simulink model "Lab1__KUKA__IIWA14_corrected"  (R2018b)
settings: Solver=ode4  StartTime=0.0  StopTime=10  FixedStep=0.001  RelTol=1e-3  EnableMultiTasking=on
values from neighbouring files (symbols this model uses):
  q0 = [pi/6; -pi/3; 0; -pi/3; -pi/6; pi/2; pi/2]    [Lab1__KUKA__IIWA14.m]
undefined symbols (not defined in the file or in its folder): v_fun, X, Y, Z
libraries: nesl_utility x41, sm_lib x27
settings Model: Creator=Ramin_hp  LastModifiedBy=Renata
settings OptimizationCC: LifeSpan=inf
settings DebuggingCC: SFUnexpectedBacktrackingDiag=warning  SFNoUnconditionalDefaultTransitionDiag=warning  SFExecutionAtInitializationDiag=none
settings SFSimCC: SimUseLocalCustomCode=off
settings RTWCC: RTWUseLocalCustomCode=off
settings CodeAppCC: StateflowObjectComments=on
settings GRTTargetCC: TargetLangStandard=C89/C90 (ANSI)  GeneratePreprocessorConditionals=Disable all
settings ConfigComp: CovMetricSettings=dw  CovHtmlReporting=on  CovSaveCumulativeToWorkspaceVar=on  CovSaveSingleToWorkspaceVar=on  CovExternalEMLEnable=off
settings SimscapeCC: SimscapeNormalizeSystem=off
settings ExplorerConfigSet: InternalSimMechanicsExplorerSettings="<ExplorerConfiguration><canonicalview>default</canonicalview><AnimationSetting><BasePlaybackSpeed>1.0</BasePlaybackSpeed><PlaybackSpeedFactor>4.0</PlaybackSpeedFactor></AnimationSetting><TilePanel><TileInfo><Tiles Columns=\"2\" Count=\"4\" Rows=\"2\"><Column Weight=\"0.5\"/><Column Weight=\"0.5\"/><Row Weight=\"0.5\"/><Row Weight=\"0.5\"/><Tile Height=\"1\" Width=\"1\" X=\"0\" Y=\"0\"/><Tile Height=\"1\" Width=\"1\" X=\"0\" Y=\"1\"/><Tile Height=\"1\" Width=\"1\" X=\"1\" Y=\"0\"/><Tile Height=\"1\" Width=\"1\" X=\"1\" Y=\"1\"/></Tiles></TileInfo><SceneInfo><SceneViewer><BGColor><R>0.60000002384185791</R><G>0.60000002384185791</G><B>0.60000002384185791</B></BGColor><Camera><DoPerspective>off</DoPerspective><Position><X>-0.162516330727092595</X><Y>-0.986821008184004533</Y><Z>0.680013463560397158</Z></Position><Center><X>-0.162516330727092595</X><Y>0.0131789918159954667</Y><Z>0.680013463560397158</Z></Center><Up><X>0</X><Y>-0</Y><Z>1</Z></Up><ViewLimDist>1</ViewLimDist><YLim>0.631454701364040472</YLim><XLim>1.11901596414291249</XLim></Camera></SceneViewer><SceneViewer><BGColor><R>0.60000002384185791</R><G>0.60000002384185791</G><B>0.60000002384185791</B></BGColor><Camera><DoPerspective>off</DoPerspective><Position><X>-0.37115316295295453</X><Y>-0.0343740496289973579</Y><Z>1.55866333636371568</Z></Position><Center><X>-0.37115316295295453</X><Y>-0.0343740496289973579</Y><Z>0.558663336363715679</Z></Center><Up><X>0</X><Y>1</Y><Z>-0</Z></Up><ViewLimDist>1</ViewLimDist><YLim>0.461610877680944443</YLim><XLim>0.818031665978841804</XLim></Camera></SceneViewer><SceneViewer><BGColor><R>0.60000002384185791</R><G>0.60000002384185791</G><B>0.60000002384185791</B></BGColor><Camera><DoPerspective>off</DoPerspective><Position><X>0.862449510483560777</X><Y>0.0193375746821874417</Y><Z>0.558663276759070793</Z></Position><Center><X>-0.137550489516439223</X><Y>0.0193375746821874417</Y><Z>0.558663276759070793</Z></Center><Up><X>-0</X><Y>0</Y><Z>1</Z></Up><ViewLimDist>1</ViewLimDist><YLim>0.575423637628555307</YLim><XLim>1.01972197730193104</XLim></Camera></SceneViewer><SceneViewer><BGColor><R>0.60000002384185791</R><G>0.60000002384185791</G><B>0.60000002384185791</B></BGColor><Camera><DoPerspective>off</DoPerspective><Position><X>0.430822299974531364</X><Y>-0.567189795663393004</Y><Z>1.10490652072727147</Z></Position><Center><X>-0.169233772465264248</X><Y>0.0328662767764026365</Y><Z>0.504850448287475606</Z></Center><Up><X>-0.408248290463863073</X><Y>0.408248290463863073</Y><Z>0.816496580927726145</Z></Up><ViewLimDist>1</ViewLimDist><YLim>0.611581102013587952</YLim><XLim>1.08379748387806174</XLim></Camera></SceneViewer></SceneInfo></TilePanel><MechEditorPanel><Cameras/><GfxPanelCameraMap/><VideoCreator><PlaybackSpeedRatio>1.0</PlaybackSpeedRatio><FrameRate>30</FrameRate><VideoFormat>Motion JPEG AVI</VideoFormat><FrameSize>auto</FrameSize></VideoCreator></MechEditorPanel></ExplorerConfiguration>"

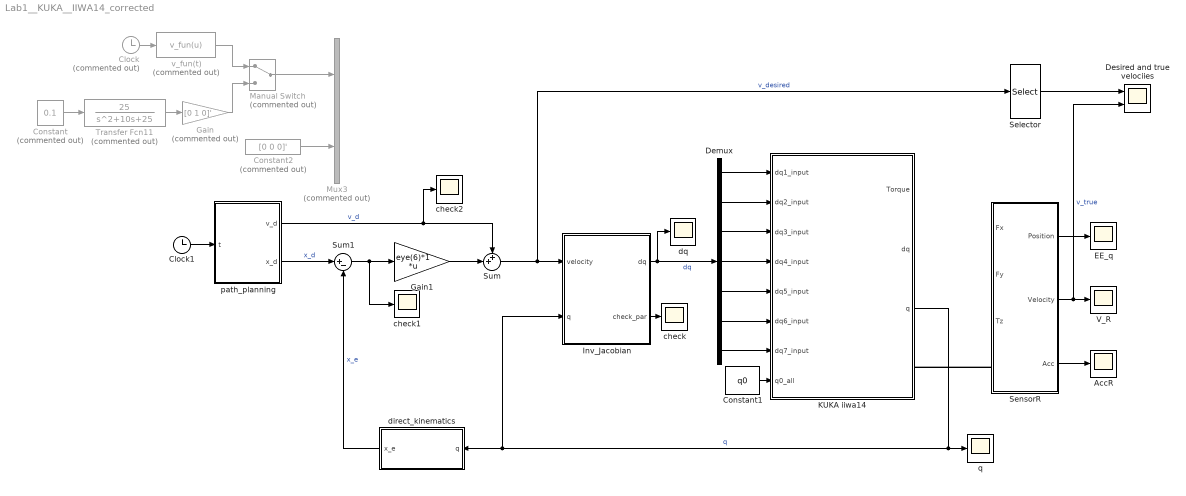
== system Lab1__KUKA__IIWA14_corrected ==
  AccR : Scope
  Clock : Clock  Commented=on
  Clock1 : Clock
  Constant : Constant  Commented=on  Value=0.1
  Constant1 : Constant  Value=q0
  Constant2 : Constant  Commented=on  Value=[0 0 0]'  VectorParams1D=off
  Demux : Demux  Outputs=7
  Desired and true velociies : Scope  NumInputPorts=2
  EE_q : Scope
  Gain : Gain  Commented=on  Gain=[0 1 0]'
  Gain1 : Gain  Gain=eye(6)*1  Multiplication=Matrix(K*u)
  Inv_Jacobian : Subsystem
  KUKA iiwa14 : Subsystem
  Manual Switch : ManualSwitch  Commented=on
  Mux3 : Mux  Commented=on  Inputs=2
  Selector : Selector  InputPortWidth=6  IndexOptions=Index vector (dialog)  Indices=[1 2 3]  OutputSizes=1
  SensorR : Subsystem
  Sum : Sum  Inputs=++|
  Sum1 : Sum  Inputs=|+-
  Transfer Fcn11 : TransferFcn  Commented=on  Numerator=[25]  Denominator=[1 10 25]
  V_R : Scope
  check : Scope
  check1 : Scope
  check2 : Scope
  direct_kinematics : MATLAB Function  TreatAsAtomicUnit=on
  dq : Scope
  path_planning : MATLAB Function  TreatAsAtomicUnit=on
  q : Scope
  v_fun(t) : MATLABFcn  Commented=on  MATLABFcn=v_fun(u)  OutputDimensions=3
  wires:
  Constant1/1 -> KUKA iiwa14/8(q0_all)
  SensorR/2(Velocity) -> Desired and true velociies/2, V_R/1  "v_true"
  SensorR/3(Acc) -> AccR/1
  SensorR/1(Position) -> EE_q/1
  Demux/5 -> KUKA iiwa14/5(dq5_input)
  Demux/4 -> KUKA iiwa14/4(dq4_input)
  Demux/6 -> KUKA iiwa14/6(dq6_input)
  Demux/1 -> KUKA iiwa14/1(dq1_input)
  Demux/2 -> KUKA iiwa14/2(dq2_input)
  Demux/3 -> KUKA iiwa14/3(dq3_input)
  path_planning/1(v_d) -> check2/1, Sum/1  "v_d"
  Demux/7 -> KUKA iiwa14/7(dq7_input)
  Inv_Jacobian/1(dq) -> Demux/1, dq/1  "dq"
  Clock/1 -> v_fun(t)/1
  v_fun(t)/1 -> Manual Switch/1
  Constant/1 -> Transfer Fcn11/1
  Constant2/1 -> Mux3/2
  Transfer Fcn11/1 -> Gain/1
  Gain/1 -> Manual Switch/2
  Manual Switch/1 -> Mux3/1
  Inv_Jacobian/2(check_par) -> check/1
  Sum/1 -> Inv_Jacobian/1(velocity), Selector/1  "v_desired"
  Gain1/1 -> Sum/2
  KUKA iiwa14/3(q) -> Inv_Jacobian/2(q), direct_kinematics/1(q), q/1  "q"
  direct_kinematics/1(x_e) -> Sum1/2  "x_e"
  Sum1/1 -> check1/1, Gain1/1
  path_planning/2(x_d) -> Sum1/1  "x_d"
  Clock1/1 -> path_planning/1(t)
  Selector/1 -> Desired and true velociies/1
  connections:
  SensorR/LConn1 -- KUKA iiwa14/RConn1

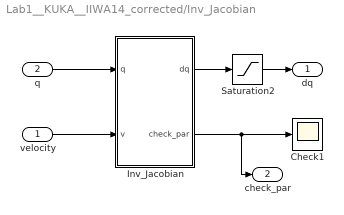
== system Lab1__KUKA__IIWA14_corrected/Inv_Jacobian ==
  velocity : Inport
  q : Inport  Port=2
  Check1 : Scope
  Inv_Jacobian : MATLAB Function  TreatAsAtomicUnit=on
  Saturation2 : Saturate  UpperLimit=9  LowerLimit=-9
  dq : Outport
  check_par : Outport  Port=2
  wires:
  velocity/1 -> Inv_Jacobian/2(v)
  q/1 -> Inv_Jacobian/1(q)
  Saturation2/1 -> dq/1
  Inv_Jacobian/1(dq) -> Saturation2/1
  Inv_Jacobian/2(check_par) -> check_par/1, Check1/1

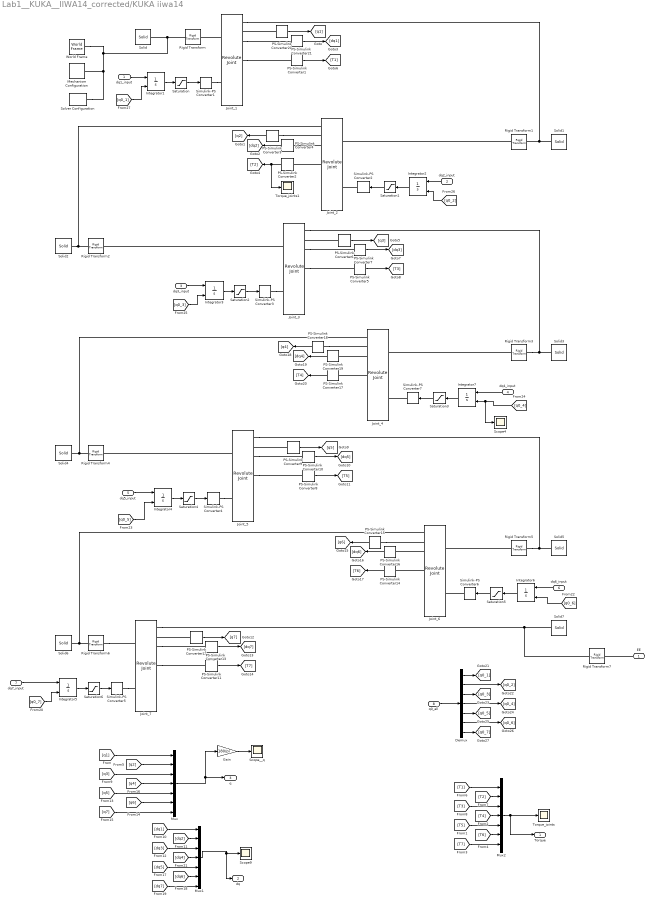
== system Lab1__KUKA__IIWA14_corrected/KUKA iiwa14 ==
  dq1_input : Inport
  dq2_input : Inport  Port=2
  dq3_input : Inport  Port=3
  dq4_input : Inport  Port=4
  dq5_input : Inport  Port=5
  dq6_input : Inport  Port=6
  dq7_input : Inport  Port=7
  q0_all : Inport  Port=8
  Demux : Demux  Outputs=7
  Gain : Gain  Gain=180/pi
  Integrator1 : Integrator  InitialConditionSource=external
  Integrator2 : Integrator  InitialConditionSource=external
  Integrator3 : Integrator  InitialConditionSource=external
  Integrator{4..7} (4 alike) : Integrator  InitialConditionSource=external  InitialCondition=90*pi/180
  Joint_{1..7} (7 alike) : sm_lib/Joints/Revolute Joint  SenseConstraintForce=on  SenseConstraintForceX=off  SenseConstraintForceY=off  SenseConstraintForceZ=off  SenseConstraintTorque=on  SenseConstraintTorqueX=off  SenseConstraintTorqueY=off  SenseConstraintTorqueZ=off  SenseTotalForce=on  SenseTotalForceX=off  SenseTotalForceY=off  SenseTotalForceZ=off  SenseTotalTorque=on  SenseTotalTorqueX=off  SenseTotalTorqueY=off  SenseTotalTorqueZ=off  CompositeWrenchDir=FollowerOnBase  CompositeWrenchFrame=BaseFrame  EquilibriumPosition=0  EquilibriumPositionUnits=deg  SpringStiffness=0  SpringStiffnessUnits=N*m/deg  DampingCoefficient=0.5  DampingCoefficientUnits=N*m/(rad/s)  TorqueActuationMode=ComputedTorque  MotionActuationMode=InputMotion  SensePosition=on  SenseVelocity=on  SenseAcceleration=on  SenseTorqueForce=on  PositionTargetSpecify=off  PositionTargetPriority=High  PositionTargetValue=0  PositionTargetValueUnits=deg  VelocityTargetSpecify=off  VelocityTargetPriority=High  VelocityTargetValue=0  VelocityTargetValueUnits=deg/s
  Mechanism Configuration : sm_lib/Utilities/Mechanism Configuration  UniformGravity=Constant  GravityVector=[0 0 -9.80665]  GravityUnits=m/s^2  LinearizationDelta=0.001
  Mux : Mux  Inputs=7
  Mux1 : Mux  Inputs=7
  Mux2 : Mux  Inputs=7
  PS-Simulink Converter{1..21} (21 alike) : nesl_utility/PS-Simulink Converter  PhysicalDomain=network_engine_domain  SubClassName=ps_output  LeftPortType=input  RightPortType=output  PseudoPeriodic=off  Frequencies=[]  Unit=1  AffineConversion=off
  Rigid Transform : sm_lib/Frames and Transforms/Rigid Transform  TranslationMethod=Cartesian  TranslationStandardOffset=0  TranslationLengthUnit=m  TranslationStandardAxis=+Z  TranslationCartesianOffset=[0 0 0.1575]  TranslationROffset=0  TranslationROffsetUnits=m  TranslationZOffset=0  TranslationZOffsetUnits=m  TranslationThetaOffset=0  TranslationThetaOffsetUnits=deg  RotationMethod=None  RotationAngleUnits=deg  RotationStandardAxis=+Z  RotationAngle=0.0  RotationArbitraryAxis=[0 0 1]  FollAlignAxisA=+X  BaseAlignAxisA=+Y  FollAlignAxisB=+Y  BaseAlignAxisB=+Z  RotationSequenceAxes=FollowerAxes  RotationSequence=XYX  RotationSequenceAngles=[0 0 0]  RotationSequenceAnglesUnits=deg  RotationMatrix=[1 0 0; 0 1 0; 0 0 1]
  Rigid Transform1 : sm_lib/Frames and Transforms/Rigid Transform  TranslationMethod=Cartesian  TranslationStandardOffset=0  TranslationLengthUnit=m  TranslationStandardAxis=+Z  TranslationCartesianOffset=[0 0 0.2025]  TranslationROffset=0  TranslationROffsetUnits=m  TranslationZOffset=0  TranslationZOffsetUnits=m  TranslationThetaOffset=0  TranslationThetaOffsetUnits=deg  RotationMethod=RotationSequence  RotationAngleUnits=deg  RotationStandardAxis=+Z  RotationAngle=0.0  RotationArbitraryAxis=[0 0 1]  FollAlignAxisA=+X  BaseAlignAxisA=+Y  FollAlignAxisB=+Y  BaseAlignAxisB=+Z  RotationSequenceAxes=BaseAxes  RotationSequence=XYZ  RotationSequenceAngles=[pi/2 0 pi]  RotationSequenceAnglesUnits=rad  RotationMatrix=[1 0 0; 0 1 0; 0 0 1]
  Rigid Transform2 : sm_lib/Frames and Transforms/Rigid Transform  TranslationMethod=Cartesian  TranslationStandardOffset=0  TranslationLengthUnit=m  TranslationStandardAxis=+Z  TranslationCartesianOffset=[0 0.2045 0]  TranslationROffset=0  TranslationROffsetUnits=m  TranslationZOffset=0  TranslationZOffsetUnits=m  TranslationThetaOffset=0  TranslationThetaOffsetUnits=deg  RotationMethod=RotationSequence  RotationAngleUnits=deg  RotationStandardAxis=+Z  RotationAngle=0.0  RotationArbitraryAxis=[0 0 1]  FollAlignAxisA=+X  BaseAlignAxisA=+Y  FollAlignAxisB=+Y  BaseAlignAxisB=+Z  RotationSequenceAxes=BaseAxes  RotationSequence=XYZ  RotationSequenceAngles=[pi/2 0 pi]  RotationSequenceAnglesUnits=rad  RotationMatrix=[1 0 0; 0 1 0; 0 0 1]
  Rigid Transform3 : sm_lib/Frames and Transforms/Rigid Transform  TranslationMethod=Cartesian  TranslationStandardOffset=0  TranslationLengthUnit=m  TranslationStandardAxis=+Z  TranslationCartesianOffset=[0 0 0.2155]  TranslationROffset=0  TranslationROffsetUnits=m  TranslationZOffset=0  TranslationZOffsetUnits=m  TranslationThetaOffset=0  TranslationThetaOffsetUnits=deg  RotationMethod=RotationSequence  RotationAngleUnits=deg  RotationStandardAxis=+Z  RotationAngle=0.0  RotationArbitraryAxis=[0 0 1]  FollAlignAxisA=+X  BaseAlignAxisA=+Y  FollAlignAxisB=+Y  BaseAlignAxisB=+Z  RotationSequenceAxes=BaseAxes  RotationSequence=XYZ  RotationSequenceAngles=[pi/2 0 0]  RotationSequenceAnglesUnits=rad  RotationMatrix=[1 0 0; 0 1 0; 0 0 1]
  Rigid Transform4 : sm_lib/Frames and Transforms/Rigid Transform  TranslationMethod=Cartesian  TranslationStandardOffset=0  TranslationLengthUnit=m  TranslationStandardAxis=+Z  TranslationCartesianOffset=[0 0.1845 0]  TranslationROffset=0  TranslationROffsetUnits=m  TranslationZOffset=0  TranslationZOffsetUnits=m  TranslationThetaOffset=0  TranslationThetaOffsetUnits=deg  RotationMethod=RotationSequence  RotationAngleUnits=deg  RotationStandardAxis=+Z  RotationAngle=0.0  RotationArbitraryAxis=[0 0 1]  FollAlignAxisA=+X  BaseAlignAxisA=+Y  FollAlignAxisB=+Y  BaseAlignAxisB=+Z  RotationSequenceAxes=BaseAxes  RotationSequence=XYZ  RotationSequenceAngles=[-pi/2 pi 0]  RotationSequenceAnglesUnits=rad  RotationMatrix=[1 0 0; 0 1 0; 0 0 1]
  Rigid Transform5 : sm_lib/Frames and Transforms/Rigid Transform  TranslationMethod=Cartesian  TranslationStandardOffset=0  TranslationLengthUnit=m  TranslationStandardAxis=+Z  TranslationCartesianOffset=[0 0 0.2155]  TranslationROffset=0  TranslationROffsetUnits=m  TranslationZOffset=0  TranslationZOffsetUnits=m  TranslationThetaOffset=0  TranslationThetaOffsetUnits=deg  RotationMethod=RotationSequence  RotationAngleUnits=deg  RotationStandardAxis=+Z  RotationAngle=0.0  RotationArbitraryAxis=[0 0 1]  FollAlignAxisA=+X  BaseAlignAxisA=+Y  FollAlignAxisB=+Y  BaseAlignAxisB=+Z  RotationSequenceAxes=BaseAxes  RotationSequence=XYZ  RotationSequenceAngles=[pi/2 0 0]  RotationSequenceAnglesUnits=rad  RotationMatrix=[1 0 0; 0 1 0; 0 0 1]
  Rigid Transform6 : sm_lib/Frames and Transforms/Rigid Transform  TranslationMethod=Cartesian  TranslationStandardOffset=0  TranslationLengthUnit=m  TranslationStandardAxis=+Z  TranslationCartesianOffset=[0 0.081 0]  TranslationROffset=0  TranslationROffsetUnits=m  TranslationZOffset=0  TranslationZOffsetUnits=m  TranslationThetaOffset=0  TranslationThetaOffsetUnits=deg  RotationMethod=RotationSequence  RotationAngleUnits=deg  RotationStandardAxis=+Z  RotationAngle=0.0  RotationArbitraryAxis=[0 0 1]  FollAlignAxisA=+X  BaseAlignAxisA=+Y  FollAlignAxisB=+Y  BaseAlignAxisB=+Z  RotationSequenceAxes=BaseAxes  RotationSequence=XYZ  RotationSequenceAngles=[-pi/2 pi 0]  RotationSequenceAnglesUnits=rad  RotationMatrix=[1 0 0; 0 1 0; 0 0 1]
  Rigid Transform7 : sm_lib/Frames and Transforms/Rigid Transform  TranslationMethod=Cartesian  TranslationStandardOffset=0  TranslationLengthUnit=m  TranslationStandardAxis=+Z  TranslationCartesianOffset=[0 0 0.05]  TranslationROffset=0  TranslationROffsetUnits=m  TranslationZOffset=0  TranslationZOffsetUnits=m  TranslationThetaOffset=0  TranslationThetaOffsetUnits=deg  RotationMethod=RotationSequence  RotationAngleUnits=deg  RotationStandardAxis=+Z  RotationAngle=0.0  RotationArbitraryAxis=[0 0 1]  FollAlignAxisA=+X  BaseAlignAxisA=+Y  FollAlignAxisB=+Y  BaseAlignAxisB=+Z  RotationSequenceAxes=BaseAxes  RotationSequence=XYZ  RotationSequenceAngles=[-pi/2 -pi/2 0]  RotationSequenceAnglesUnits=rad  RotationMatrix=[1 0 0; 0 1 0; 0 0 1]
  Saturation : Saturate  UpperLimit=170*pi/180  LowerLimit=-170*pi/180
  Saturation1 : Saturate  UpperLimit=120*pi/180  LowerLimit=-120*pi/180
  Saturation2 : Saturate  UpperLimit=170*pi/180  LowerLimit=-170*pi/180
  Saturation3 : Saturate  UpperLimit=120*pi/180  LowerLimit=-120*pi/180
  Saturation4 : Saturate  UpperLimit=170*pi/180  LowerLimit=-170*pi/180
  Saturation5 : Saturate  UpperLimit=120*pi/180  LowerLimit=-120*pi/180
  Saturation6 : Saturate  UpperLimit=175*pi/180  LowerLimit=-175*pi/180
  Scope4 : Scope
  Scope9 : Scope
  Scope__q : Scope
  Simulink-PS Converter{1..7} (7 alike) : nesl_utility/Simulink-PS Converter  PhysicalDomain=network_engine_domain  SubClassName=ps_input  LeftPortType=input  RightPortType=output  PseudoPeriodic=off  Frequencies=[]  NoiseDistribution=none  NoiseParameters=[]  Unit=1  AffineConversion=off  FilteringAndDerivatives=filter  SimscapeFilterOrder=2  InputFilterTimeConstant=0.01  UdotUserProvided=1
  Solid : sm_lib/Body Elements/Solid  InertiaType=Custom  Mass=5  MassUnits=kg  CenterOfMass=[-0.1 0 0.07]  CenterOfMassUnits=m  MomentsOfInertia=[0.05 0.06 0.03]  MomentsOfInertiaUnits=kg*m^2  ProductsOfInertia=[0 0 0]  ProductsOfInertiaUnits=kg*m^2  BasedOnType=Mass  Density=1500  DensityUnits=kg/(m^3)  DoExposeReferenceFrame=on  SerializedFrames=<Frames/>  GraphicType=FromGeometry  MarkerShape=Sphere  MarkerSize=10  GraphicVisPropType=SimpleVisualProperties  GraphicDiffuseColor=[0.4 0.4 0.4]  GraphicSpecularColor=[0.5 0.5 0.5 1.0]  GraphicAmbientColor=[0.15 0.15 0.15 1.0]  GraphicEmissiveColor=[0.0 0.0 0.0 1.0]  GraphicShininess=75  GraphicOpacity=1.0  GeometryShape=FromFile  RectangleSize=[1 1]  RectangleSizeUnits=m  BrickDimensions=[1 0.1 0.1]  BrickDimensionUnits=m  CylinderRadius=1  CylinderRadiusUnits=m  CylinderLength=1  CylinderLengthUnits=m  SphereRadius=1  SphereRadiusUnits=m  EllipsoidRadii=[1 1 1]  EllipsoidRadiiUnits=m  ExtrusionCrossSection=[1 1; -1 1; -1 -1; 1 -1]  ExtrusionCrossSectionUnits=m  ExtrusionLength=1  ExtrusionLengthUnits=m  PolygonNumSides=3  PolygonOuterRadius=1  PolygonOuterRadiusUnits=m  ExtGeomFileType=STL  ExtGeomFileName=.\iiwa14_visual\link_0.stl  ExtGeomFileUnits=m  RevolutionCrossSection=[1 1; 1 -1; 2 -1; 2 1]  RevolutionCrossSectionUnits=m  RevolutionExtent=Full  RevolutionAngle=180  RevolutionAngleUnits=deg
  Solid1 : sm_lib/Body Elements/Solid  InertiaType=Custom  Mass=4  MassUnits=kg  CenterOfMass=[0 -0.03 0.12]  CenterOfMassUnits=m  MomentsOfInertia=[0.1 0.09 0.02]  MomentsOfInertiaUnits=kg*m^2  ProductsOfInertia=[0 0 0]  ProductsOfInertiaUnits=kg*m^2  BasedOnType=Mass  Density=1500  DensityUnits=kg/(m^3)  DoExposeReferenceFrame=on  SerializedFrames=<Frames/>  GraphicType=FromGeometry  MarkerShape=Sphere  MarkerSize=10  GraphicVisPropType=SimpleVisualProperties  GraphicDiffuseColor=[255/255 108/255 10/255]  GraphicSpecularColor=[0.5 0.5 0.5 1.0]  GraphicAmbientColor=[0.15 0.15 0.15 1.0]  GraphicEmissiveColor=[0.0 0.0 0.0 1.0]  GraphicShininess=75  GraphicOpacity=1.0  GeometryShape=FromFile  RectangleSize=[1 1]  RectangleSizeUnits=m  BrickDimensions=[1 0.1 0.1]  BrickDimensionUnits=m  CylinderRadius=1  CylinderRadiusUnits=m  CylinderLength=1  CylinderLengthUnits=m  SphereRadius=1  SphereRadiusUnits=m  EllipsoidRadii=[1 1 1]  EllipsoidRadiiUnits=m  ExtrusionCrossSection=[1 1; -1 1; -1 -1; 1 -1]  ExtrusionCrossSectionUnits=m  ExtrusionLength=1  ExtrusionLengthUnits=m  PolygonNumSides=3  PolygonOuterRadius=1  PolygonOuterRadiusUnits=m  ExtGeomFileType=STL  ExtGeomFileName=.\iiwa14_visual\link_1.stl  ExtGeomFileUnits=m  RevolutionCrossSection=[1 1; 1 -1; 2 -1; 2 1]  RevolutionCrossSectionUnits=m  RevolutionExtent=Full  RevolutionAngle=180  RevolutionAngleUnits=deg
  Solid2 : sm_lib/Body Elements/Solid  InertiaType=Custom  Mass=4  MassUnits=kg  CenterOfMass=[0.0003 0.059 0.042]  CenterOfMassUnits=m  MomentsOfInertia=[0.05 0.018 0.044]  MomentsOfInertiaUnits=kg*m^2  ProductsOfInertia=[0 0 0]  ProductsOfInertiaUnits=kg*m^2  BasedOnType=Mass  Density=1500  DensityUnits=kg/(m^3)  DoExposeReferenceFrame=on  SerializedFrames=<Frames/>  GraphicType=FromGeometry  MarkerShape=Sphere  MarkerSize=10  GraphicVisPropType=SimpleVisualProperties  GraphicDiffuseColor=[255/255 108/255 10/255]  GraphicSpecularColor=[0.5 0.5 0.5 1.0]  GraphicAmbientColor=[0.15 0.15 0.15 1.0]  GraphicEmissiveColor=[0.0 0.0 0.0 1.0]  GraphicShininess=75  GraphicOpacity=1.0  GeometryShape=FromFile  RectangleSize=[1 1]  RectangleSizeUnits=m  BrickDimensions=[1 0.1 0.1]  BrickDimensionUnits=m  CylinderRadius=1  CylinderRadiusUnits=m  CylinderLength=1  CylinderLengthUnits=m  SphereRadius=1  SphereRadiusUnits=m  EllipsoidRadii=[1 1 1]  EllipsoidRadiiUnits=m  ExtrusionCrossSection=[1 1; -1 1; -1 -1; 1 -1]  ExtrusionCrossSectionUnits=m  ExtrusionLength=1  ExtrusionLengthUnits=m  PolygonNumSides=3  PolygonOuterRadius=1  PolygonOuterRadiusUnits=m  ExtGeomFileType=STL  ExtGeomFileName=.\iiwa14_visual\link_2.stl  ExtGeomFileUnits=m  RevolutionCrossSection=[1 1; 1 -1; 2 -1; 2 1]  RevolutionCrossSectionUnits=m  RevolutionExtent=Full  RevolutionAngle=180  RevolutionAngleUnits=deg
  Solid3 : sm_lib/Body Elements/Solid  InertiaType=Custom  Mass=3  MassUnits=kg  CenterOfMass=[0 0.03 0.13]  CenterOfMassUnits=m  MomentsOfInertia=[0.08 0.075 0.01]  MomentsOfInertiaUnits=kg*m^2  ProductsOfInertia=[0 0 0]  ProductsOfInertiaUnits=kg*m^2  BasedOnType=Mass  Density=1500  DensityUnits=kg/(m^3)  DoExposeReferenceFrame=on  SerializedFrames=<Frames/>  GraphicType=FromGeometry  MarkerShape=Sphere  MarkerSize=10  GraphicVisPropType=SimpleVisualProperties  GraphicDiffuseColor=[255/255 108/255 10/255]  GraphicSpecularColor=[0.5 0.5 0.5 1.0]  GraphicAmbientColor=[0.15 0.15 0.15 1.0]  GraphicEmissiveColor=[0.0 0.0 0.0 1.0]  GraphicShininess=75  GraphicOpacity=1.0  GeometryShape=FromFile  RectangleSize=[1 1]  RectangleSizeUnits=m  BrickDimensions=[1 0.1 0.1]  BrickDimensionUnits=m  CylinderRadius=1  CylinderRadiusUnits=m  CylinderLength=1  CylinderLengthUnits=m  SphereRadius=1  SphereRadiusUnits=m  EllipsoidRadii=[1 1 1]  EllipsoidRadiiUnits=m  ExtrusionCrossSection=[1 1; -1 1; -1 -1; 1 -1]  ExtrusionCrossSectionUnits=m  ExtrusionLength=1  ExtrusionLengthUnits=m  PolygonNumSides=3  PolygonOuterRadius=1  PolygonOuterRadiusUnits=m  ExtGeomFileType=STL  ExtGeomFileName=.\iiwa14_visual\link_3.stl  ExtGeomFileUnits=m  RevolutionCrossSection=[1 1; 1 -1; 2 -1; 2 1]  RevolutionCrossSectionUnits=m  RevolutionExtent=Full  RevolutionAngle=180  RevolutionAngleUnits=deg
  Solid4 : sm_lib/Body Elements/Solid  InertiaType=Custom  Mass=2.7  MassUnits=kg  CenterOfMass=[0 0.067 0.034]  CenterOfMassUnits=m  MomentsOfInertia="[0.03  0.01  0.029]"  MomentsOfInertiaUnits=kg*m^2  ProductsOfInertia=[0 0 0]  ProductsOfInertiaUnits=kg*m^2  BasedOnType=Mass  Density=1500  DensityUnits=kg/(m^3)  DoExposeReferenceFrame=on  SerializedFrames=<Frames/>  GraphicType=FromGeometry  MarkerShape=Sphere  MarkerSize=10  GraphicVisPropType=SimpleVisualProperties  GraphicDiffuseColor=[255/255 108/255 10/255]  GraphicSpecularColor=[0.5 0.5 0.5 1.0]  GraphicAmbientColor=[0.15 0.15 0.15 1.0]  GraphicEmissiveColor=[0.0 0.0 0.0 1.0]  GraphicShininess=75  GraphicOpacity=1.0  GeometryShape=FromFile  RectangleSize=[1 1]  RectangleSizeUnits=m  BrickDimensions=[1 0.1 0.1]  BrickDimensionUnits=m  CylinderRadius=1  CylinderRadiusUnits=m  CylinderLength=1  CylinderLengthUnits=m  SphereRadius=1  SphereRadiusUnits=m  EllipsoidRadii=[1 1 1]  EllipsoidRadiiUnits=m  ExtrusionCrossSection=[1 1; -1 1; -1 -1; 1 -1]  ExtrusionCrossSectionUnits=m  ExtrusionLength=1  ExtrusionLengthUnits=m  PolygonNumSides=3  PolygonOuterRadius=1  PolygonOuterRadiusUnits=m  ExtGeomFileType=STL  ExtGeomFileName=.\iiwa14_visual\link_4.stl  ExtGeomFileUnits=m  RevolutionCrossSection=[1 1; 1 -1; 2 -1; 2 1]  RevolutionCrossSectionUnits=m  RevolutionExtent=Full  RevolutionAngle=180  RevolutionAngleUnits=deg
  Solid5 : sm_lib/Body Elements/Solid  InertiaType=Custom  Mass=1.7  MassUnits=kg  CenterOfMass=[0.0001 0.021 0.076]  CenterOfMassUnits=m  MomentsOfInertia=[0.02 0.018 0.005]  MomentsOfInertiaUnits=kg*m^2  ProductsOfInertia=[0 0 0]  ProductsOfInertiaUnits=kg*m^2  BasedOnType=Mass  Density=1500  DensityUnits=kg/(m^3)  DoExposeReferenceFrame=on  SerializedFrames=<Frames/>  GraphicType=FromGeometry  MarkerShape=Sphere  MarkerSize=10  GraphicVisPropType=SimpleVisualProperties  GraphicDiffuseColor=[255/255 108/255 10/255]  GraphicSpecularColor=[0.5 0.5 0.5 1.0]  GraphicAmbientColor=[0.15 0.15 0.15 1.0]  GraphicEmissiveColor=[0.0 0.0 0.0 1.0]  GraphicShininess=75  GraphicOpacity=1.0  GeometryShape=FromFile  RectangleSize=[1 1]  RectangleSizeUnits=m  BrickDimensions=[1 0.1 0.1]  BrickDimensionUnits=m  CylinderRadius=1  CylinderRadiusUnits=m  CylinderLength=1  CylinderLengthUnits=m  SphereRadius=1  SphereRadiusUnits=m  EllipsoidRadii=[1 1 1]  EllipsoidRadiiUnits=m  ExtrusionCrossSection=[1 1; -1 1; -1 -1; 1 -1]  ExtrusionCrossSectionUnits=m  ExtrusionLength=1  ExtrusionLengthUnits=m  PolygonNumSides=3  PolygonOuterRadius=1  PolygonOuterRadiusUnits=m  ExtGeomFileType=STL  ExtGeomFileName=.\iiwa14_visual\link_5.stl  ExtGeomFileUnits=m  RevolutionCrossSection=[1 1; 1 -1; 2 -1; 2 1]  RevolutionCrossSectionUnits=m  RevolutionExtent=Full  RevolutionAngle=180  RevolutionAngleUnits=deg
  Solid6 : sm_lib/Body Elements/Solid  InertiaType=Custom  Mass=1.8  MassUnits=kg  CenterOfMass=[0 0.0006 0.0004]  CenterOfMassUnits=m  MomentsOfInertia=[0.005 0.0036 0.0047]  MomentsOfInertiaUnits=kg*m^2  ProductsOfInertia=[0 0 0]  ProductsOfInertiaUnits=kg*m^2  BasedOnType=Mass  Density=1500  DensityUnits=kg/(m^3)  DoExposeReferenceFrame=on  SerializedFrames=<Frames/>  GraphicType=FromGeometry  MarkerShape=Sphere  MarkerSize=10  GraphicVisPropType=SimpleVisualProperties  GraphicDiffuseColor=[255/255 108/255 10/255]  GraphicSpecularColor=[0.5 0.5 0.5 1.0]  GraphicAmbientColor=[0.15 0.15 0.15 1.0]  GraphicEmissiveColor=[0.0 0.0 0.0 1.0]  GraphicShininess=75  GraphicOpacity=1.0  GeometryShape=FromFile  RectangleSize=[1 1]  RectangleSizeUnits=m  BrickDimensions=[1 0.1 0.1]  BrickDimensionUnits=m  CylinderRadius=1  CylinderRadiusUnits=m  CylinderLength=1  CylinderLengthUnits=m  SphereRadius=1  SphereRadiusUnits=m  EllipsoidRadii=[1 1 1]  EllipsoidRadiiUnits=m  ExtrusionCrossSection=[1 1; -1 1; -1 -1; 1 -1]  ExtrusionCrossSectionUnits=m  ExtrusionLength=1  ExtrusionLengthUnits=m  PolygonNumSides=3  PolygonOuterRadius=1  PolygonOuterRadiusUnits=m  ExtGeomFileType=STL  ExtGeomFileName=.\iiwa14_visual\link_6.stl  ExtGeomFileUnits=m  RevolutionCrossSection=[1 1; 1 -1; 2 -1; 2 1]  RevolutionCrossSectionUnits=m  RevolutionExtent=Full  RevolutionAngle=180  RevolutionAngleUnits=deg
  Solid7 : sm_lib/Body Elements/Solid  InertiaType=Custom  Mass=0.3  MassUnits=kg  CenterOfMass=[0 0 0.02]  CenterOfMassUnits=m  MomentsOfInertia=[0.001 0.001 0.001]  MomentsOfInertiaUnits=kg*m^2  ProductsOfInertia=[0 0 0]  ProductsOfInertiaUnits=kg*m^2  BasedOnType=Mass  Density=1500  DensityUnits=kg/(m^3)  DoExposeReferenceFrame=on  SerializedFrames=<Frames/>  GraphicType=FromGeometry  MarkerShape=Sphere  MarkerSize=10  GraphicVisPropType=SimpleVisualProperties  GraphicDiffuseColor=[0.4 0.4 0.4]  GraphicSpecularColor=[0.5 0.5 0.5 1.0]  GraphicAmbientColor=[0.15 0.15 0.15 1.0]  GraphicEmissiveColor=[0.0 0.0 0.0 1.0]  GraphicShininess=75  GraphicOpacity=1.0  GeometryShape=FromFile  RectangleSize=[1 1]  RectangleSizeUnits=m  BrickDimensions=[1 0.1 0.1]  BrickDimensionUnits=m  CylinderRadius=1  CylinderRadiusUnits=m  CylinderLength=1  CylinderLengthUnits=m  SphereRadius=1  SphereRadiusUnits=m  EllipsoidRadii=[1 1 1]  EllipsoidRadiiUnits=m  ExtrusionCrossSection=[1 1; -1 1; -1 -1; 1 -1]  ExtrusionCrossSectionUnits=m  ExtrusionLength=1  ExtrusionLengthUnits=m  PolygonNumSides=3  PolygonOuterRadius=1  PolygonOuterRadiusUnits=m  ExtGeomFileType=STL  ExtGeomFileName=.\iiwa14_visual\link_7.stl  ExtGeomFileUnits=m  RevolutionCrossSection=[1 1; 1 -1; 2 -1; 2 1]  RevolutionCrossSectionUnits=m  RevolutionExtent=Full  RevolutionAngle=180  RevolutionAngleUnits=deg
  Solver Configuration : nesl_utility/Solver Configuration  PhysicalDomain=network_engine_domain  SubClassName=solver  LeftPortType=input  RightPortType=generic  Tones=[]  Harmonics=[]  SimulateNoise=off  Profile=off  UseLocalSampling=off  EnableSwitchedLinearOptims=on  FrequencyDomain=off  UseCCode=off  RelTol=0.001  AbsTol=1e-06  MinStep=1e-09  ToWorkspace=off  RevertToSquareIcSolve=off  NumHomotopyIterations=100  PhasorMode=off  PhasorModeNumHarmonics=1  DoDC=off  ResidualTolerance=1e-09  UseLocalSolver=off  LocalSolverChoice=NE_BACKWARD_EULER_ADVANCER  LocalSolverSampleTime=0.001  DoFixedCost=off  MaxNonlinIter=3  MaxModeIter=2  LinearAlgebra=Sparse  EquationFormulation=NE_TIME_EF  DelaysMemoryBudget=1024  AutomaticFiltering=on  FilteringTimeConstant=0.001  PartitionStorageMethod=AS_NEEDED  PartitionMemoryBudget=1024
  Torque_joints : Scope
  Torque_joints1 : Scope
  World Frame : sm_lib/Frames and Transforms/World Frame
  EE : PMIOPort  Side=Right
  Torque : Outport
  dq : Outport  Port=2
  q : Outport  Port=3
  wires:
  dq1_input/1 -> Integrator1/1
  Integrator1/1 -> Saturation/1
  PS-Simulink Converter20/1 -> [q1]
  PS-Simulink Converter21/1 -> [dq1]
  PS-Simulink Converter1/1 -> [T1]
  dq2_input/1 -> Integrator2/1
  Integrator2/1 -> Saturation1/1
  PS-Simulink Converter3/1 -> [q2]
  PS-Simulink Converter4/1 -> [dq2]
  PS-Simulink Converter2/1 -> Torque_joints1/1, [T2]
  dq3_input/1 -> Integrator3/1
  Integrator3/1 -> Saturation2/1
  PS-Simulink Converter6/1 -> [q3]
  PS-Simulink Converter7/1 -> [dq3]
  PS-Simulink Converter5/1 -> [T3]
  dq5_input/1 -> Integrator4/1
  Integrator4/1 -> Saturation4/1
  PS-Simulink Converter9/1 -> [q5]
  PS-Simulink Converter10/1 -> [dq5]
  PS-Simulink Converter8/1 -> [T5]
  dq7_input/1 -> Integrator5/1
  Integrator5/1 -> Saturation6/1
  PS-Simulink Converter12/1 -> [q7]
  PS-Simulink Converter13/1 -> [dq7]
  PS-Simulink Converter11/1 -> [T7]
  dq6_input/1 -> Integrator6/1
  Integrator6/1 -> Saturation5/1
  PS-Simulink Converter15/1 -> [q6]
  PS-Simulink Converter16/1 -> [dq6]
  PS-Simulink Converter14/1 -> [T6]
  dq4_input/1 -> Integrator7/1
  Integrator7/1 -> Saturation3/1
  PS-Simulink Converter18/1 -> [q4]
  PS-Simulink Converter19/1 -> [dq4]
  PS-Simulink Converter17/1 -> [T4]
  Mux2/1 -> Torque/1, Torque_joints/1
  [T1] -> Mux2/1
  [T3] -> Mux2/3
  [T2] -> Mux2/2
  [T5] -> Mux2/5
  [T7] -> Mux2/7
  [T4] -> Mux2/4
  [T6] -> Mux2/6
  Mux1/1 -> dq/1, Scope9/1
  Mux/1 -> Gain/1, q/1
  [q1] -> Mux/1
  [q2] -> Mux/2
  [q3] -> Mux/3
  [dq1] -> Mux1/1
  [dq3] -> Mux1/3
  [dq2] -> Mux1/2
  Gain/1 -> Scope__q/1
  [q5] -> Mux/5
  [q7] -> Mux/7
  [q4] -> Mux/4
  [q6] -> Mux/6
  [dq5] -> Mux1/5
  [dq7] -> Mux1/7
  [dq6] -> Mux1/6
  [dq4] -> Mux1/4
  Saturation/1 -> Simulink-PS Converter1/1
  Saturation1/1 -> Simulink-PS Converter2/1
  Saturation2/1 -> Simulink-PS Converter3/1
  Saturation3/1 -> Simulink-PS Converter7/1
  Saturation4/1 -> Simulink-PS Converter4/1
  Saturation5/1 -> Simulink-PS Converter6/1
  Saturation6/1 -> Simulink-PS Converter5/1
  q0_all/1 -> Demux/1
  Demux/3 -> [q0_3]
  Demux/5 -> [q0_5]
  Demux/7 -> [q0_7]
  Demux/1 -> [q0_1]
  Demux/4 -> [q0_4]
  Demux/6 -> [q0_6]
  Demux/2 -> [q0_2]
  [q0_7] -> Integrator5/2
  [q0_6] -> Integrator6/2
  [q0_5] -> Integrator4/2
  [q0_4] -> Scope4/1, Integrator7/2
  [q0_3] -> Integrator3/2
  [q0_2] -> Integrator2/2
  [q0_1] -> Integrator1/2
  connections:
  Mechanism Configuration/RConn1 -- Solver Configuration/RConn1 -- World Frame/RConn1 -- Rigid Transform/LConn1 -- Solid/RConn1
  Rigid Transform1/LConn1 -- Joint_1/RConn1 -- Solid1/RConn1
  Solid2/RConn1 -- Rigid Transform2/LConn1 -- Joint_2/RConn1
  Rigid Transform3/LConn1 -- Joint_3/RConn1 -- Solid3/RConn1
  Rigid Transform4/LConn1 -- Joint_4/RConn1 -- Solid4/RConn1
  Rigid Transform5/LConn1 -- Joint_5/RConn1 -- Solid5/RConn1
  Rigid Transform6/LConn1 -- Joint_6/RConn1 -- Solid6/RConn1
  Rigid Transform5/RConn1 -- Joint_6/LConn1
  Simulink-PS Converter7/RConn1 -- Joint_4/LConn2
  Simulink-PS Converter1/RConn1 -- Joint_1/LConn2
  PS-Simulink Converter3/LConn1 -- Joint_2/RConn2
  PS-Simulink Converter15/LConn1 -- Joint_6/RConn2
  Joint_2/RConn3 -- PS-Simulink Converter4/LConn1
  Simulink-PS Converter3/RConn1 -- Joint_3/LConn2
  Joint_6/RConn3 -- PS-Simulink Converter16/LConn1
  Rigid Transform6/RConn1 -- Joint_7/LConn1
  Simulink-PS Converter2/RConn1 -- Joint_2/LConn2
  Joint_5/RConn5 -- PS-Simulink Converter8/LConn1
  Simulink-PS Converter4/RConn1 -- Joint_5/LConn2
  PS-Simulink Converter9/LConn1 -- Joint_5/RConn2
  Rigid Transform1/RConn1 -- Joint_2/LConn1
  PS-Simulink Converter6/LConn1 -- Joint_3/RConn2
  PS-Simulink Converter20/LConn1 -- Joint_1/RConn2
  Joint_1/LConn1 -- Rigid Transform/RConn1
  Joint_1/RConn3 -- PS-Simulink Converter21/LConn1
  PS-Simulink Converter18/LConn1 -- Joint_4/RConn2
  Simulink-PS Converter6/RConn1 -- Joint_6/LConn2
  Joint_4/RConn3 -- PS-Simulink Converter19/LConn1
  Joint_3/RConn5 -- PS-Simulink Converter5/LConn1
  Simulink-PS Converter5/RConn1 -- Joint_7/LConn2
  Joint_6/RConn5 -- PS-Simulink Converter14/LConn1
  PS-Simulink Converter12/LConn1 -- Joint_7/RConn2
  Joint_7/RConn5 -- PS-Simulink Converter11/LConn1
  Joint_7/RConn3 -- PS-Simulink Converter13/LConn1
  Joint_5/LConn1 -- Rigid Transform4/RConn1
  Rigid Transform3/RConn1 -- Joint_4/LConn1
  Joint_3/LConn1 -- Rigid Transform2/RConn1
  Joint_3/RConn3 -- PS-Simulink Converter7/LConn1
  Joint_4/RConn5 -- PS-Simulink Converter17/LConn1
  Joint_2/RConn5 -- PS-Simulink Converter2/LConn1
  Joint_5/RConn3 -- PS-Simulink Converter10/LConn1
  Joint_1/RConn5 -- PS-Simulink Converter1/LConn1
  Joint_7/RConn1 -- Rigid Transform7/LConn1 -- Solid7/RConn1
  EE/RConn1 -- Rigid Transform7/RConn1

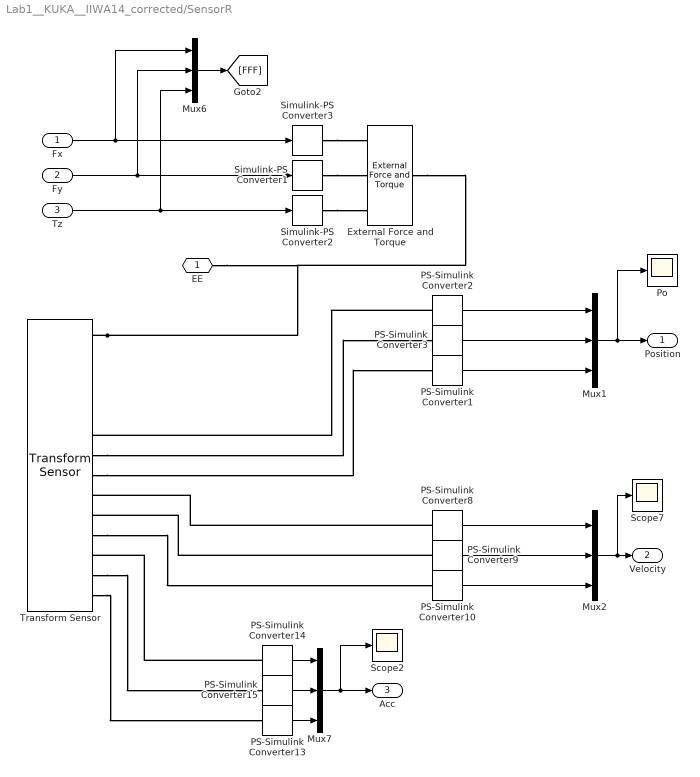
== system Lab1__KUKA__IIWA14_corrected/SensorR ==
  Fx : Inport
  Fy : Inport  Port=2
  Tz : Inport  Port=3
  External Force and Torque : sm_lib/Forces and Torques/External Force and Torque  ForceResolutionFrame=World  EnableForceX=on  EnableForceY=on  EnableForceZ=off  EnableForce=off  TorqueResolutionFrame=World  EnableTorqueX=off  EnableTorqueY=off  EnableTorqueZ=on  EnableTorque=off
  Mux{1..2,6..7} (4 alike) : Mux  Inputs=3
  PS-Simulink Converter{1..3,8..10,13..15} (9 alike) : nesl_utility/PS-Simulink Converter  PhysicalDomain=network_engine_domain  SubClassName=ps_output  LeftPortType=input  RightPortType=output  PseudoPeriodic=off  Frequencies=[]  Unit=1  AffineConversion=off
  Po : Scope
  Scope2 : Scope
  Scope7 : Scope
  Simulink-PS Converter1 : nesl_utility/Simulink-PS Converter  PhysicalDomain=network_engine_domain  SubClassName=ps_input  LeftPortType=input  RightPortType=output  PseudoPeriodic=off  Frequencies=[]  NoiseDistribution=none  NoiseParameters=[]  Unit=1  AffineConversion=off  FilteringAndDerivatives=zero  SimscapeFilterOrder=1  InputFilterTimeConstant=0.001  UdotUserProvided=1
  Simulink-PS Converter2 : nesl_utility/Simulink-PS Converter  PhysicalDomain=network_engine_domain  SubClassName=ps_input  LeftPortType=input  RightPortType=output  PseudoPeriodic=off  Frequencies=[]  NoiseDistribution=none  NoiseParameters=[]  Unit=1  AffineConversion=off  FilteringAndDerivatives=zero  SimscapeFilterOrder=1  InputFilterTimeConstant=0.001  UdotUserProvided=1
  Simulink-PS Converter3 : nesl_utility/Simulink-PS Converter  PhysicalDomain=network_engine_domain  SubClassName=ps_input  LeftPortType=input  RightPortType=output  PseudoPeriodic=off  Frequencies=[]  NoiseDistribution=none  NoiseParameters=[]  Unit=1  AffineConversion=off  FilteringAndDerivatives=zero  SimscapeFilterOrder=1  InputFilterTimeConstant=0.001  UdotUserProvided=1
  Transform Sensor : sm_lib/Frames and Transforms/Transform Sensor  MeasurementFrame=World  SenseAngle=on  SenseAxis=on  SenseAngle1=off  SenseAngle2=off  SenseAngle3=off  SenseQ=off  SenseR=off  SenseOmegaX=off  SenseOmegaY=off  SenseOmegaZ=on  SenseOmega1=off  SenseOmega2=off  SenseOmega3=off  SenseQDot=off  SenseRDot=off  SenseAlphaX=off  SenseAlphaY=off  SenseAlphaZ=on  SenseAlpha1=off  SenseAlpha2=off  SenseAlpha3=off  SenseQDDot=off  SenseRDDot=off  SenseX=on  SenseY=on  SenseZ=on  SenseRad=off  SenseAzim=off  SenseDist=off  SenseInc=off  SenseXDot=on  SenseYDot=on  SenseZDot=on  SenseRadDot=off  SenseAzimDot=off  SenseDistDot=off  SenseIncDot=off  SenseXDDot=on  SenseYDDot=on  SenseZDDot=on  SenseRadDDot=off  SenseAzimDDot=off  SenseDistDDot=off  SenseIncDDot=off
  EE : PMIOPort  Side=Left
  Position : Outport
  Velocity : Outport  Port=2
  Acc : Outport  Port=3
  wires:
  Mux2/1 -> Scope7/1, Velocity/1
  PS-Simulink Converter10/1 -> Mux2/3
  PS-Simulink Converter8/1 -> Mux2/1
  Mux1/1 -> Position/1, Po/1
  PS-Simulink Converter1/1 -> Mux1/3
  PS-Simulink Converter2/1 -> Mux1/1
  PS-Simulink Converter3/1 -> Mux1/2
  Fx/1 -> Mux6/1, Simulink-PS Converter3/1
  Fy/1 -> Mux6/2, Simulink-PS Converter1/1
  Tz/1 -> Mux6/3, Simulink-PS Converter2/1
  PS-Simulink Converter9/1 -> Mux2/2
  Mux6/1 -> [FFF]
  PS-Simulink Converter13/1 -> Mux7/3
  PS-Simulink Converter14/1 -> Mux7/1
  PS-Simulink Converter15/1 -> Mux7/2
  Mux7/1 -> Acc/1, Scope2/1
  connections:
  Transform Sensor/RConn1 -- External Force and Torque/RConn1 -- EE/RConn1
  PS-Simulink Converter2/LConn1 -- Transform Sensor/RConn6
  Transform Sensor/RConn7 -- PS-Simulink Converter3/LConn1
  Transform Sensor/RConn13 -- PS-Simulink Converter15/LConn1
  PS-Simulink Converter9/LConn1 -- Transform Sensor/RConn10
  PS-Simulink Converter8/LConn1 -- Transform Sensor/RConn9
  Simulink-PS Converter3/RConn1 -- External Force and Torque/LConn1
  Simulink-PS Converter1/RConn1 -- External Force and Torque/LConn2
  Simulink-PS Converter2/RConn1 -- External Force and Torque/LConn3
  PS-Simulink Converter14/LConn1 -- Transform Sensor/RConn12
  Transform Sensor/RConn8 -- PS-Simulink Converter1/LConn1
  Transform Sensor/RConn11 -- PS-Simulink Converter10/LConn1
  Transform Sensor/RConn14 -- PS-Simulink Converter13/LConn1

== matlab function Lab1__KUKA__IIWA14_corrected/Inv_Jacobian/Inv_Jacobian ==
  data: q input; v input; dq output; check_par output
function [dq,check_par] = Inv_Jacobian(q,v)

% dq = zeros(6,1);
% J = zeros(6,7);
dq = zeros(7,1);

J_geom = Jacobian_KUKA7(q);

T_0_e = KUKA_FKin(q);
eulZYZ = rotm2eul(T_0_e(1:3,1:3),'ZYZ');

J_analyt = rb.T_zyz2geom(eulZYZ) \ J_geom;

% dq = J_analyt \ v;
dq = J_analyt(1:3,:) \ v(1:3);

check_par = min(svd(J_analyt)) ;%< 1e-4;

== matlab function Lab1__KUKA__IIWA14_corrected/direct_kinematics ==
  data: q input; x_e output
function x_e = direct_kinematics(q)

T_0_e = KUKA_FKin(q);
eulZYZ = rotm2eul(T_0_e(1:3,1:3),'ZYZ')';

x_e = [T_0_e(1:3,4);
       eulZYZ];

== matlab function Lab1__KUKA__IIWA14_corrected/path_planning ==
  data: t input; v_d output; x_d output
function [v_d,x_d] = path_planning(t)

%% Question 4a

% x_d = [0;%.1*t;
%        0;
%        0;
%        0;
%        0
%        0];
%    
% v_d = [0;%.1;
%        0;
%        0;
%        0;
%        0;
%        0];


%% Question 4b

x_d = [-0.2;
       -0.0008*t^3+0.012*t^2-0.2;
       1;
       0;
       0;
       0]

v_d = [0;
      (3*t)/125 - (3*t^2)/1250;
       0;
       0;
       0;
       0];
